simulink model "GraphicalFunction2_2018a"  (R2018a)
settings: Solver=VariableStepAuto  StartTime=0.0  StopTime=0.1  RelTol=1e-3
settings Model: Creator=86188  LastModifiedBy=bzhan

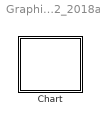
== system GraphicalFunction2_2018a ==
  Chart : Stateflow chart  TreatAsAtomicUnit=on

== stateflow chart GraphicalFunction2_2018a/Chart ==
  state i=set(sn) [function]
    (junction 10) -> (junction 4) : {a(i)=b(i);i = i + 1;f("set")}
    (junction 3) -> (junction 10) [order 1] : [i<=sn]
    (junction 4) -> (junction 3)
    (default) -> (junction 3) : {i=1;}
    (junction 3) -> (junction 9) [order 2]
  state A
    en: f("en_A");
    data=set(3);
  state B
    en: f("en_B");g()
  (default) -> A
  A -> B
  data: sn function_input; i function_output; s function_input; b local double size=[1 5] =[100 200 300 400 500]; a local double size=[1 5] =[0 0 0 0 0]; data local
  function f(s):
    | function f(s)
    |   fprintf(s+"\n");
  function g:
    | function g
    |   fprintf("%.0f %.0f %.0f %.0f %.0f\n", a(1), a(2), a(3), a(4), a(5));
